simulink model "singl_phase_inverter_with_pwm_without"  (R2020a)
settings: Solver=VariableStepAuto  StartTime=0.0  StopTime=1  RelTol=1e-3
libraries: powerlib x49, simulink x3, powerlib_meascontrol x3
settings Model: Creator=hp  LastModifiedBy=hp

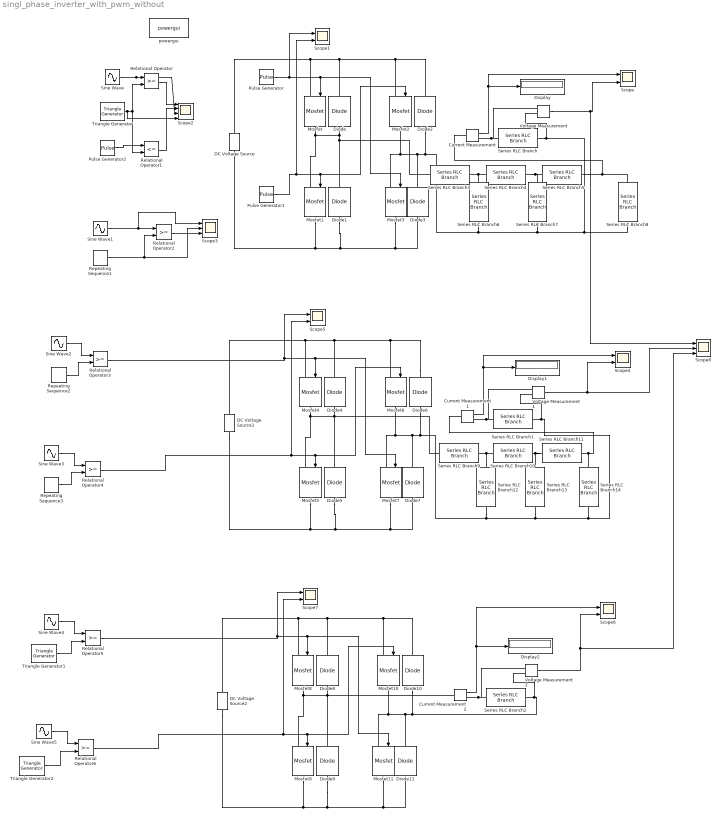
== system singl_phase_inverter_with_pwm_without ==
  Current Measurement : powerlib/Measurements/Current Measurement  PhasorSimulation=off  OutputType=Complex  PSBequivalent=0
  Current Measurement1 : powerlib/Measurements/Current Measurement  PhasorSimulation=off  OutputType=Complex  PSBequivalent=0
  Current Measurement2 : powerlib/Measurements/Current Measurement  PhasorSimulation=off  OutputType=Complex  PSBequivalent=0
  DC Voltage Source : powerlib/Electrical Sources/DC Voltage Source  Amplitude=100  Measurements=None
  DC Voltage Source1 : powerlib/Electrical Sources/DC Voltage Source  Amplitude=100  Measurements=None
  DC Voltage Source2 : powerlib/Electrical Sources/DC Voltage Source  Amplitude=100  Measurements=None
  Diode{,1..11} (12 alike) : powerlib/Power Electronics/Diode  Ron=0.001  Lon=0  Vf=0.8  IC=0  UseSnubber=0  Rs=500  Cs=250e-9  Measurements=off
  Display : Display
  Display1 : Display
  Display2 : Display
  Mosfet{,1..11} (12 alike) : powerlib/Power Electronics/Mosfet  Ron=0.1  Lon=0  Rd=0.01  Vfd=0  IC=0  Rs=1e5  Cs=inf  Measurements=off
  Pulse Generator : DiscretePulseGenerator  PulseType=Time based  Period=1/50  PulseWidth=50
  Pulse Generator1 : DiscretePulseGenerator  PulseType=Time based  Period=1/50  PulseWidth=50  PhaseDelay=180/(360*50)
  Pulse Generator2 : DiscretePulseGenerator  PulseType=Time based  Period=1/50  PulseWidth=50
  Relational Operator{,2..6} (6 alike) : RelationalOperator  OutDataTypeStr=boolean  RndMeth=Simplest
  Relational Operator1 : RelationalOperator  Operator=<=  OutDataTypeStr=boolean  RndMeth=Simplest
  Repeating Sequence1 : simulink/Sources/Repeating Sequence  rep_seq_t=[0 .0005 .001]  rep_seq_y=[0 1 0]
  Repeating Sequence2 : simulink/Sources/Repeating Sequence  rep_seq_t=[0 .0005 .001]  rep_seq_y=[0 1 0]
  Repeating Sequence3 : simulink/Sources/Repeating Sequence  rep_seq_t=[0 .0005 .001]  rep_seq_y=[0 1 0]
  Scope{,1,4..7} (6 alike) : Scope  NumInputPorts=2
  Scope2 : Scope  NumInputPorts=4
  Scope3 : Scope  NumInputPorts=3
  Scope8 : Scope  NumInputPorts=3
  Series RLC Branch : powerlib/Elements/Series RLC Branch  LConnTagsString=__new0  RConnTagsString=__new0  BranchType=R  Resistance=10  Inductance=1e-3  SetiL0=off  InitialCurrent=0  Capacitance=1e-6  Setx0=off  InitialVoltage=0  Measurements=None
  Series RLC Branch1 : powerlib/Elements/Series RLC Branch  LConnTagsString=__new0  RConnTagsString=__new0  BranchType=R  Resistance=10  Inductance=1e-3  SetiL0=off  InitialCurrent=0  Capacitance=1e-6  Setx0=off  InitialVoltage=0  Measurements=None
  Series RLC Branch{3..5,9..11} (6 alike) : powerlib/Elements/Series RLC Branch  LConnTagsString=__new0  RConnTagsString=__new0  BranchType=R  Resistance=1  Inductance=1e-3  SetiL0=off  InitialCurrent=0  Capacitance=1e-6  Setx0=off  InitialVoltage=0  Measurements=None
  Series RLC Branch{6..8,12..14} (6 alike) : powerlib/Elements/Series RLC Branch  LConnTagsString=__new0  RConnTagsString=__new0  BranchType=C  Resistance=10  Inductance=1e-3  SetiL0=off  InitialCurrent=0  Capacitance=3.183e-3  Setx0=off  InitialVoltage=0  Measurements=None
  Series RLC Branch2 : powerlib/Elements/Series RLC Branch  LConnTagsString=__new0  RConnTagsString=__new0  BranchType=R  Resistance=10  Inductance=1e-3  SetiL0=off  InitialCurrent=0  Capacitance=1e-6  Setx0=off  InitialVoltage=0  Measurements=None
  Sine Wave{,1..2,4} (4 alike) : Sin  Frequency=2*pi*50  SampleTime=0
  Sine Wave3 : Sin  Frequency=2*pi*50  Phase=pi  SampleTime=0
  Sine Wave5 : Sin  Frequency=2*pi*50  Phase=pi  SampleTime=0
  Triangle Generator : powerlib_meascontrol/Pulse & Signal Generators/Triangle Generator  Freq=5e2  Phase=90  Ts=0
  Triangle Generator1 : powerlib_meascontrol/Pulse & Signal Generators/Triangle Generator  Freq=5e2  Phase=90  Ts=0
  Triangle Generator2 : powerlib_meascontrol/Pulse & Signal Generators/Triangle Generator  Freq=5e2  Phase=90  Ts=0
  Voltage Measurement : powerlib/Measurements/Voltage Measurement  PhasorSimulation=off  OutputType=Complex  PSBequivalent=0
  Voltage Measurement1 : powerlib/Measurements/Voltage Measurement  PhasorSimulation=off  OutputType=Complex  PSBequivalent=0
  Voltage Measurement2 : powerlib/Measurements/Voltage Measurement  PhasorSimulation=off  OutputType=Complex  PSBequivalent=0
  powergui : powerlib/powergui  Priority=1  SimulationMode=Discrete  SampleTime=50e-6  frequency=60  Iterations=50  frequencyindice=0  Pbase=100e6  ErrMax=1e-4  UnitsV=kV  UnitsW=MW  buscounter=0  FunctionMessages=off  echomessages=off  EnableUseOfTLC=off  CurrentSourceSwitches=off  DisableSnubberDevices=off  DisableRonSwitches=off  DisableVfSwitches=off  DisplayEquations=off  AutomaticDiscreteSolvers=off  SolverType=Tustin/Backward Euler (TBE)  Interpol=off  ExternalGateDelay=off  methode=off  Ts=100  x0status=blocks  SPID=on  SwTol=0  HookPort=off  NonlinearTolerance=1e-4  nMaxIteration=100  ContinueOnMaxIteration=off  RestoreLinks=warning  ResistiveCurrentMeasurement=off  Frange=[0:2:500]  Ylog=off  Xlog=on  ShowGrid=off  save=off  variable=ZData  structure=0  ZoomFFT=off  StartTime=0.0  cycles=1  DisplayStyle=1  fundamental=60  FreqAxis=off  MaxFrequency=1000  frequencyindicesteady=1  RmsSteady=1  display=off
  wires:
  Current Measurement/1 -> Display/1, Scope/1
  Pulse Generator/1 -> Scope1/1, Mosfet3/1, Mosfet/1
  Pulse Generator1/1 -> Scope1/2, Mosfet2/1, Mosfet1/1
  Voltage Measurement/1 -> Scope8/1, Scope/2
  Triangle Generator/1 -> Scope2/4, Relational Operator1/2, Relational Operator/2
  Pulse Generator2/1 -> Relational Operator1/1
  Relational Operator/1 -> Scope2/1
  Relational Operator1/1 -> Scope2/2
  Sine Wave/1 -> Scope2/3, Relational Operator/1
  Sine Wave1/1 -> Scope3/1, Relational Operator2/1
  Repeating Sequence1/1 -> Scope3/2, Relational Operator2/2
  Relational Operator2/1 -> Scope3/3
  Current Measurement1/1 -> Display1/1, Scope4/1
  Relational Operator4/1 -> Scope5/2, Mosfet6/1, Mosfet5/1
  Voltage Measurement1/1 -> Scope8/2, Scope4/2
  Relational Operator3/1 -> Scope5/1, Mosfet7/1, Mosfet4/1
  Sine Wave2/1 -> Relational Operator3/1
  Repeating Sequence2/1 -> Relational Operator3/2
  Sine Wave3/1 -> Relational Operator4/1
  Repeating Sequence3/1 -> Relational Operator4/2
  Triangle Generator2/1 -> Relational Operator6/2
  Current Measurement2/1 -> Display2/1, Scope6/1
  Relational Operator5/1 -> Scope7/1, Mosfet11/1, Mosfet8/1
  Triangle Generator1/1 -> Relational Operator5/2
  Sine Wave5/1 -> Relational Operator6/1
  Sine Wave4/1 -> Relational Operator5/1
  Voltage Measurement2/1 -> Scope8/3, Scope6/2
  Relational Operator6/1 -> Scope7/2, Mosfet10/1, Mosfet9/1
  connections:
  DC Voltage Source/RConn1 -- Mosfet/LConn1 -- Mosfet2/LConn1 -- Diode2/RConn1 -- Diode/RConn1
  DC Voltage Source/LConn1 -- Diode1/LConn1 -- Mosfet3/RConn1 -- Diode3/LConn1 -- Mosfet1/RConn1
  Mosfet/RConn1 -- Series RLC Branch3/LConn1 -- Diode1/RConn1 -- Diode/LConn1 -- Mosfet1/LConn1
  Series RLC Branch/RConn1 -- Series RLC Branch6/RConn1 -- Mosfet3/LConn1 -- Mosfet2/RConn1 -- Diode3/RConn1 -- Diode2/LConn1 -- Series RLC Branch7/RConn1 -- Series RLC Branch8/RConn1 -- Voltage Measurement/LConn2
  Series RLC Branch/LConn1 -- Current Measurement/RConn1 -- Voltage Measurement/LConn1
  Diode5/RConn1 -- Series RLC Branch9/LConn1 -- Mosfet4/RConn1 -- Mosfet5/LConn1 -- Diode4/LConn1
  Diode7/LConn1 -- Mosfet7/RConn1 -- DC Voltage Source1/LConn1 -- Mosfet5/RConn1 -- Diode5/LConn1
  Diode6/RConn1 -- DC Voltage Source1/RConn1 -- Mosfet4/LConn1 -- Diode4/RConn1 -- Mosfet6/LConn1
  Voltage Measurement1/LConn1 -- Series RLC Branch1/LConn1 -- Current Measurement1/RConn1
  Diode10/LConn1 -- Series RLC Branch2/RConn1 -- Voltage Measurement2/LConn2 -- Mosfet11/LConn1 -- Mosfet10/RConn1 -- Diode11/RConn1
  Diode9/LConn1 -- Diode11/LConn1 -- Mosfet11/RConn1 -- DC Voltage Source2/LConn1 -- Mosfet9/RConn1
  Mosfet8/LConn1 -- Diode10/RConn1 -- Mosfet10/LConn1 -- Diode8/RConn1 -- DC Voltage Source2/RConn1
  Current Measurement2/RConn1 -- Voltage Measurement2/LConn1 -- Series RLC Branch2/LConn1
  Mosfet9/LConn1 -- Diode9/RConn1 -- Diode8/LConn1 -- Current Measurement2/LConn1 -- Mosfet8/RConn1
  Series RLC Branch6/LConn1 -- Series RLC Branch4/LConn1 -- Series RLC Branch3/RConn1
  Series RLC Branch4/RConn1 -- Series RLC Branch7/LConn1 -- Series RLC Branch5/LConn1
  Series RLC Branch8/LConn1 -- Series RLC Branch5/RConn1 -- Current Measurement/LConn1
  Series RLC Branch10/RConn1 -- Series RLC Branch13/LConn1 -- Series RLC Branch11/LConn1
  Series RLC Branch9/RConn1 -- Series RLC Branch12/LConn1 -- Series RLC Branch10/LConn1
  Series RLC Branch1/RConn1 -- Voltage Measurement1/LConn2 -- Series RLC Branch13/RConn1 -- Series RLC Branch12/RConn1 -- Mosfet7/LConn1 -- Mosfet6/RConn1 -- Diode7/RConn1 -- Diode6/LConn1 -- Series RLC Branch14/RConn1
  Series RLC Branch14/LConn1 -- Current Measurement1/LConn1 -- Series RLC Branch11/RConn1
